simulink model "sosanhvlntdtblackbox"  (R2022a)
settings: Solver=VariableStepAuto  StartTime=0.0  StopTime=10.0  RelTol=1e-3
libraries: arduinolib x2
settings Model: Creator=TUAN  LastModifiedBy=TUAN

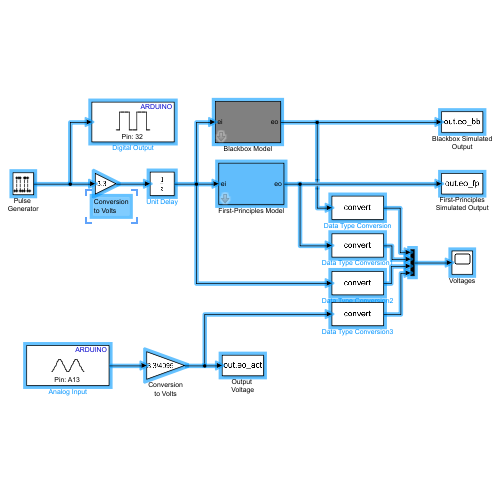
[thumbnail: Simulink's stored preview of the top-level diagram]
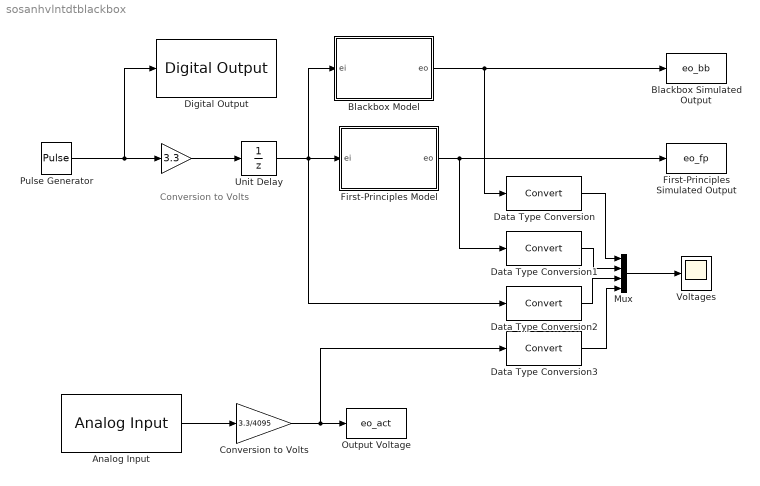
== system sosanhvlntdtblackbox ==
  note: Conversion
      | to Volts
  " " : Gain  Gain=3.3
  Analog Input : arduinolib/Analog Input  pinNumber=13  ReadResultsOnly=off  ConversionTriggerSource=Software  ExternalTriggerType=uint32( 0 )  OutputDataType=uint16  EnableConversionCompleteNotify=off  EnableOuputStatus=off  SampleTime=-1  blockPlatform=arduino
  Blackbox Model : Subsystem  mask{K=1, tau=1.15}
      mask prompts: K "DC gain"; tau "Time constant"
      mask Display:
      | port_label('input',1,'ei')
      | port_label('output',1,'eo')
  Blackbox Simulated Output : ToWorkspace  VariableName=eo_bb  SampleTime=-1
      settings: Save2DSignal=2-D array (concatenate along first dimension)
  Conversion to Volts : Gain  Gain=3.3/4095
  Data Type Conversion{,1..3} (4 alike) : DataTypeConversion  SaturateOnIntegerOverflow=off  RndMeth=Floor
  Digital Output : arduinolib/Digital Output  pinNumber=32  Direction=output  blockPlatform=arduino
  First-Principles Simulated Output : ToWorkspace  VariableName=eo_fp  SampleTime=-1
      settings: Save2DSignal=2-D array (concatenate along first dimension)
  First-Principles Model : Subsystem  mask{R=1000000, C=1*10^-6, q_init=0}
      mask prompts: R "Resistance"; C "Capacitance"; q_init "Initial charge on capacitor"
      mask Display:
      | port_label('input',1,'ei')
      | port_label('output',1,'eo')
  Mux : Mux
  Output Voltage : ToWorkspace  VariableName=eo_act  SampleTime=-1
      settings: Save2DSignal=2-D array (concatenate along first dimension)
  Pulse Generator : DiscretePulseGenerator  Period=100  PulseWidth=50  SampleTime=0.1
  Unit Delay : UnitDelay  SampleTime=-1  HasFrameUpgradeWarning=on
  Voltages : Scope
  wires:
  First-Principles Model/1(eo) -> Data Type Conversion1/1, First-Principles Simulated Output/1
  Blackbox Model/1(eo) -> Data Type Conversion/1, Blackbox Simulated Output/1
  Unit Delay/1 -> Data Type Conversion2/1, Blackbox Model/1(ei), First-Principles Model/1(ei)
  Analog Input/1 -> Conversion to Volts/1
  Pulse Generator/1 -> " "/1, Digital Output/1
  Conversion to Volts/1 -> Data Type Conversion3/1, Output Voltage/1
  Data Type Conversion/1 -> Mux/1
  " "/1 -> Unit Delay/1
  Data Type Conversion3/1 -> Mux/4
  Mux/1 -> Voltages/1
  Data Type Conversion2/1 -> Mux/3
  Data Type Conversion1/1 -> Mux/2

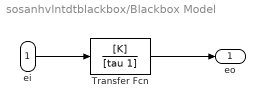
== system sosanhvlntdtblackbox/Blackbox Model ==
  ei : Inport
  Transfer Fcn : TransferFcn  Numerator=[K]  Denominator=[tau 1]
  eo : Outport  VectorParamsAs1DForOutWhenUnconnected=off
  wires:
  ei/1 -> Transfer Fcn/1
  Transfer Fcn/1 -> eo/1

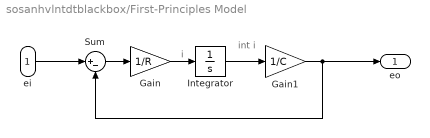
== system sosanhvlntdtblackbox/First-Principles Model ==
  note: int i
  note: i
  ei : Inport
  Gain : Gain  Gain=1/R  SampleTime=0.1
  Gain1 : Gain  Gain=1/C  SampleTime=0.1
  Integrator : Integrator  InitialCondition=q_init
  Sum : Sum  Inputs=|+-
  eo : Outport  VectorParamsAs1DForOutWhenUnconnected=off
  wires:
  Gain/1 -> Integrator/1
  Sum/1 -> Gain/1
  Integrator/1 -> Gain1/1
  Gain1/1 -> Sum/2, eo/1
  ei/1 -> Sum/1
